simulink model "Lab_5"  (Simulink 9.2)
settings: Solver=VariableStepAuto  StartTime=0.0  StopTime=simulation_time  MaxStep=0.1
values from neighbouring files (symbols this model uses):
  a = (r_a + r_p)/2    (= 7178)    [main.m]
  A_BN_0 = eye(3)    [main.m]
  A_i = [A_i_1, A_i_2, A_i_3]    [main.m]
  alpha_m = deg2rad(11)    [main.m]
  C_d = 2.2    [main.m]
  dim = [w, l, h]    [main.m]
  epsilon = deg2rad(23.439)    [main.m]
  i = 40    [main.m]
  I = [I_1,   0,  0 ... (first row only)    [main.m]
  I_inv = inv(I)    [main.m]
  k_d = -0.001    [main.m]
  k_p = -0.001    [main.m]
  m_m = (a_m^3*H_0)*(4*pi/mu_0)    [main.m]
  mu = 398600    [main.m]
  n = 2*pi/(60*60*24*365)    (= 1.99238499086e-07)    [main.m]
  nadir_vector = [1; 0; 0]    [main.m]
  OMG = 0    [main.m]
  omg = 0    [main.m]
  phi_0 = 0    [main.m]
  psi_0 = 0    [main.m]
  Q_C = [ q_c(4)  q_c(3)  -q_c(2) -q_c(1) ... (first row only)    [main.m]
  R_e = 6.378e+03    (= 6378)    [main.m]
  rho_d = 0.1    [main.m]
  rho_s = 0.5    [main.m]
  theta = 0    [main.m]
  theta_0 = 0    [main.m]
  w_0 = [w1_0,w2_0,w3_0]    [main.m]
  w_e = [0 0 0.00007291]    [main.m]
undefined symbols (not defined in the file or in its folder): q_0
libraries: sharedtransform x2, vrlib x2, sharedutil x2
settings Model: Creator=fcuzzocrea  LastModifiedBy=fcuzzocrea
settings DataIOCC: LimitDataPoints=off  SaveFormat=Dataset  SignalLoggingSaveFormat=Dataset
settings OptimizationCC: LifeSpan=auto
settings DebuggingCC: UnderspecifiedInitializationDetection=Simplified  MergeDetectMultiDrivingBlocksExec=error  FcnCallInpInsideContextMsg=error  StateNameClashWarn=none  LibraryContextMissingDiagnostic=none  SFUnexpectedBacktrackingDiag=error  SFNoUnconditionalDefaultTransitionDiag=error  SFExecutionAtInitializationDiag=warning
settings HardwareCC: ProdBitPerPointer=64  ProdBitPerSizeT=64  ProdBitPerPtrDiffT=64  ProdLargestAtomicFloat=Float  ProdIntDivRoundTo=Zero  ProdEndianess=LittleEndian  ProdWordSize=64  ProdHWDeviceType=Intel->x86-64 (Windows64)
settings ModelReferenceCC: PropagateSignalLabelsOutOfModel=on
settings CodeAppCC: StateflowObjectComments=off
settings GRTTargetCC: TargetLangStandard=C99 (ISO)  GeneratePreprocessorConditionals=Use local settings  CombineOutputUpdateFcns=on  GRTInterface=off
settings ConfigComp: CovMetricSettings=dwe  CovHtmlReporting=off  CovSaveCumulativeToWorkspaceVar=off  CovSaveSingleToWorkspaceVar=off  CovExternalEMLEnable=on

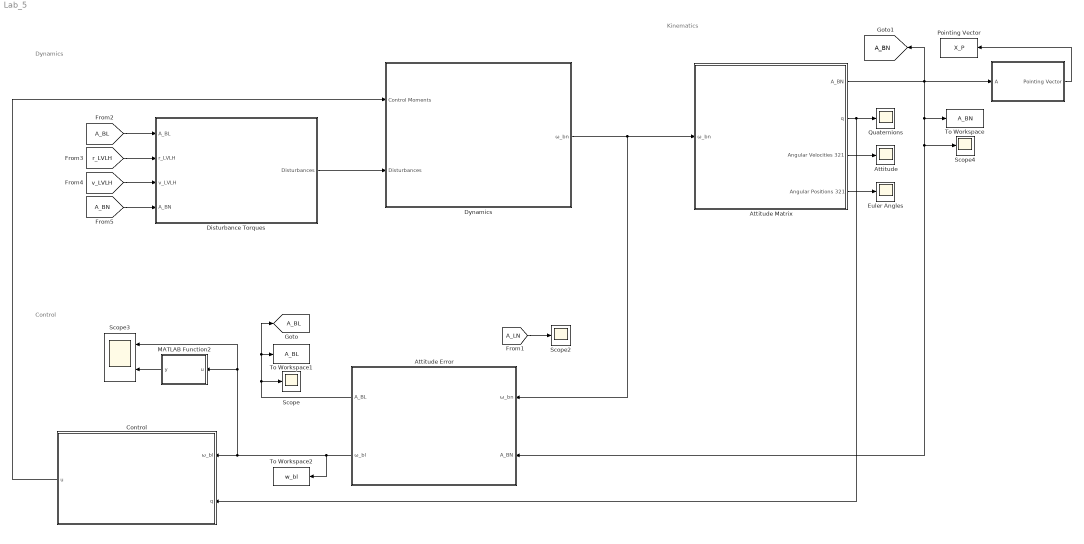
== system Lab_5 ==
  note: Dynamics
  note: Kinematics
  note: Control
  " " : Subsystem
  Attitude : Scope
  Attitude Error : Subsystem
  Attitude Matrix : Subsystem
  Control : Subsystem
  Disturbance Torques : Subsystem
  "Dynamics  " : Subsystem
  Euler Angles : Scope
  MATLAB Function2 : MATLAB Function  TreatAsAtomicUnit=on
  Pointing Vector : ToWorkspace  VariableName=X_P  SampleTime=-1
  Quaternions : Scope
  Scope : Scope
  Scope2 : Scope
  Scope3 : Scope  NumInputPorts=2
  Scope4 : Scope
  To Workspace : ToWorkspace  VariableName=A_BN  SampleTime=-1
  To Workspace1 : ToWorkspace  VariableName=A_BL  SampleTime=-1
  To Workspace2 : ToWorkspace  VariableName=w_bl  SampleTime=-1
  tag scope: A_BL=global, A_BN=global
  wires:
  Disturbance Torques/1(Disturbances) -> "Dynamics  "/2("Disturbances ")
  [r_LVLH] -> Disturbance Torques/2(r_LVLH)
  Attitude Error/1(A_BL) -> [A_BL], To Workspace1/1, Scope/1
  [A_BN] -> Disturbance Torques/4(A_BN)
  Control/1(u) -> "Dynamics  "/1(Control Moments)
  [A_BL] -> Disturbance Torques/1(A_BL)
  " "/1("Pointing Vector ") -> Pointing Vector/1
  Attitude Matrix/3(Angular Velocities 321) -> Attitude/1
  MATLAB Function2/1(y) -> Scope3/2
  [v_LVLH] -> Disturbance Torques/3(v_LVLH)
  Attitude Matrix/2(q) -> Quaternions/1, Control/2(q)
  Attitude Matrix/4(Angular Positions 321) -> Euler Angles/1
  [A_LN] -> Scope2/1
  Attitude Error/2(ω_bl) -> Control/1(ω_bl), Scope3/1, MATLAB Function2/1(u), To Workspace2/1
  Attitude Matrix/1(A_BN) -> Scope4/1, Attitude Error/2(A_BN), To Workspace/1, " "/1(A), [A_BN]
  "Dynamics  "/1(ω_bn) -> Attitude Error/1(ω_bn), Attitude Matrix/1(ω_bn)

== system Lab_5/  ==
  A : Inport
  Constant3 : Constant  Value=[1; 0; 0]  VectorParams1D=off
  Math Function : Math  Operator=transpose  SaturateOnIntegerOverflow=on
  Product1 : Product  Multiplication=Matrix(*)
  "Pointing Vector " : Outport
  wires:
  Constant3/1 -> Product1/2
  Math Function/1 -> Product1/1
  A/1 -> Math Function/1
  Product1/1 -> "Pointing Vector "/1

== system Lab_5/Attitude Error ==
  ω_bn : Inport
  A_BN : Inport  Port=2
  Angular velocity of the  orbital pointing  frame : Subsystem
  Attitude Error : Subsystem
  Body\LVLH Difference : Subsystem
  A_BL : Outport
  ω_bl : Outport  Port=2
  wires:
  ω_bn/1 -> Attitude Error/1(ω_bn)
  A_BN/1 -> Body\LVLH Difference/1("A_BN ")
  Body\LVLH Difference/1("A_BL   ") -> A_BL/1, Attitude Error/2("A_BL ")
  Angular velocity of the  orbital pointing  frame/1(ω_ln) -> Attitude Error/3("ω_ln ")
  Attitude Error/1(ω_bl) -> ω_bl/1

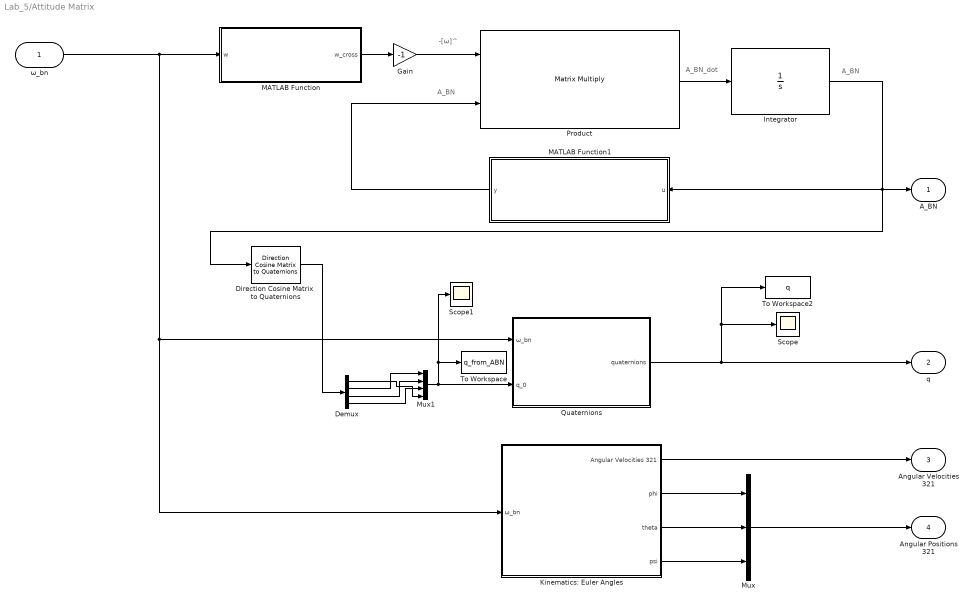
== system Lab_5/Attitude Matrix ==
  note: -[ω]^
  note: A_BN_dot
  note: A_BN
  note: A_BN
  ω_bn : Inport  Unit=rad/s  PortDimensions=3
  Demux : Demux
  Direction Cosine Matrix  to Quaternions : sharedtransform/Direction Cosine Matrix  to Quaternions  aMode=0  action=None  tolerance=eps(2)
      settings: SourceProductName=Aerospace Blockset  SourceProductBaseCode=AE
  Gain : Gain  Gain=-1
  Integrator : Integrator  InitialCondition=A_BN_0
  Kinematics: Euler Angles : Subsystem
  MATLAB Function : MATLAB Function  TreatAsAtomicUnit=on
  MATLAB Function1 : MATLAB Function  TreatAsAtomicUnit=on
  Mux : Mux  Inputs=3
  Mux1 : Mux
  Product : Product  Multiplication=Matrix(*)
  Quaternions : Subsystem
  Scope : Scope
  Scope1 : Scope
  To Workspace : ToWorkspace  VariableName=q_from_ABN  SampleTime=-1
  To Workspace2 : ToWorkspace  VariableName=q  SampleTime=-1
  A_BN : Outport
  q : Outport  Port=2
  Angular Velocities 321 : Outport  Port=3
  Angular Positions 321 : Outport  Port=4
  wires:
  Product/1 -> Integrator/1
  Integrator/1 -> MATLAB Function1/1(u), Direction Cosine Matrix  to Quaternions/1, A_BN/1
  MATLAB Function/1(w_cross) -> Gain/1
  MATLAB Function1/1(y) -> Product/2
  ω_bn/1 -> Quaternions/1(ω_bn), Kinematics: Euler Angles/1(ω_bn), MATLAB Function/1(w)
  Kinematics: Euler Angles/1(Angular Velocities 321) -> Angular Velocities 321/1
  Kinematics: Euler Angles/3(theta) -> Mux/2
  Mux/1 -> Angular Positions 321/1
  Kinematics: Euler Angles/4(psi) -> Mux/3
  Kinematics: Euler Angles/2(phi) -> Mux/1
  Gain/1 -> Product/1
  Mux1/1 -> Quaternions/2("q_0 "), To Workspace/1, Scope1/1
  Quaternions/1(quaternions) -> q/1, Scope/1, To Workspace2/1
  Demux/1 -> Mux1/4
  Demux/2 -> Mux1/1
  Demux/3 -> Mux1/2
  Demux/4 -> Mux1/3
  Direction Cosine Matrix  to Quaternions/1 -> Demux/1

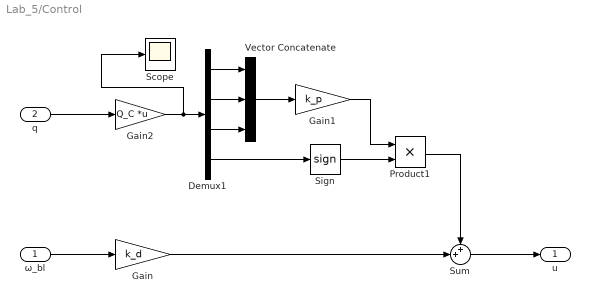
== system Lab_5/Control ==
  ω_bl : Inport
  q : Inport  Port=2
  Demux1 : Demux
  Gain : Gain  Gain=k_d
  Gain1 : Gain  Gain=k_p
  Gain2 : Gain  Gain=Q_C  Multiplication=Matrix(K*u)
  Product1 : Product
  Scope : Scope
  Sign : Signum
  Sum : Sum  Inputs=++|
  Vector Concatenate : Concatenate  NumInputs=3
  u : Outport
  wires:
  ω_bl/1 -> Gain/1
  q/1 -> Gain2/1
  Sum/1 -> u/1
  Demux1/4 -> Sign/1
  Demux1/1 -> Vector Concatenate/1
  Demux1/2 -> Vector Concatenate/2
  Demux1/3 -> Vector Concatenate/3
  Vector Concatenate/1 -> Gain1/1
  Gain1/1 -> Product1/1
  Sign/1 -> Product1/2
  Product1/1 -> Sum/1
  Gain/1 -> Sum/2
  Gain2/1 -> Scope/1, Demux1/1

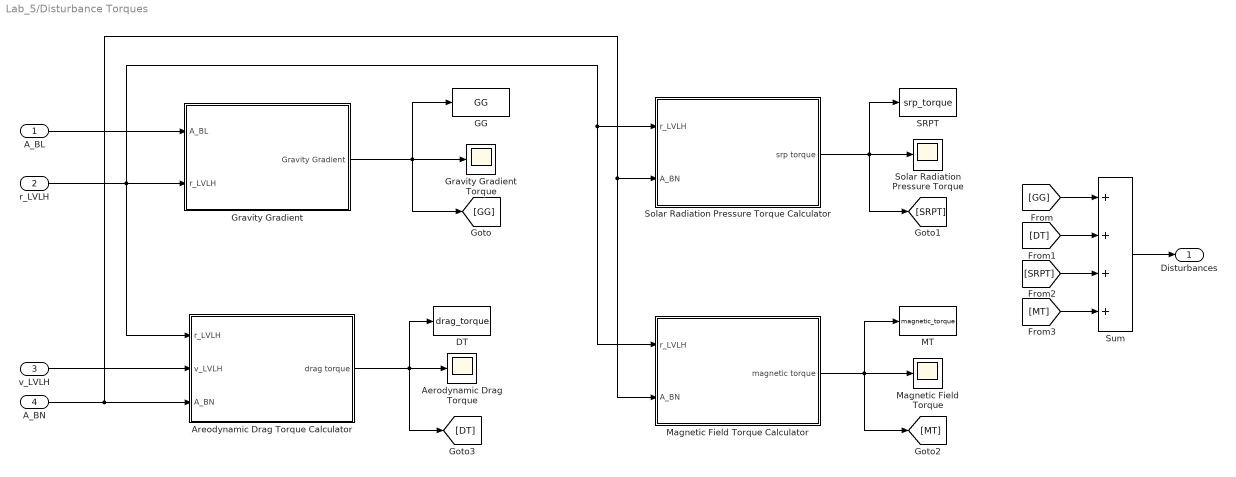
== system Lab_5/Disturbance Torques ==
  A_BL : Inport
  r_LVLH : Inport  Port=2
  v_LVLH : Inport  Port=3
  A_BN : Inport  Port=4
  Aerodynamic Drag Torque : Scope
  "Areodynamic Drag Torque Calculator " : Subsystem
  DT : ToWorkspace  VariableName=drag_torque  SampleTime=-1
  GG : ToWorkspace  VariableName=GG  SampleTime=-1
  Gravity Gradient : Subsystem
  "Gravity Gradient Torque " : Scope
  MT : ToWorkspace  VariableName=magnetic_torque  SampleTime=-1
  Magnetic Field Torque : Scope
  Magnetic Field Torque Calculator : Subsystem
  SRPT : ToWorkspace  VariableName=srp_torque  SampleTime=-1
  Solar Radiation Pressure Torque : Scope
  Solar Radiation Pressure Torque Calculator : Subsystem
  Sum : Sum  Inputs=++++
  Disturbances : Outport
  wires:
  A_BL/1 -> Gravity Gradient/1(A_BL)
  Gravity Gradient/1(Gravity Gradient) -> GG/1, "Gravity Gradient Torque "/1, [GG]
  v_LVLH/1 -> "Areodynamic Drag Torque Calculator "/2(v_LVLH)
  A_BN/1 -> Magnetic Field Torque Calculator/2(A_BN), Solar Radiation Pressure Torque Calculator/2(A_BN), "Areodynamic Drag Torque Calculator "/3(A_BN)
  "Areodynamic Drag Torque Calculator "/1("drag torque ") -> [DT], DT/1, Aerodynamic Drag Torque/1
  Solar Radiation Pressure Torque Calculator/1("srp torque ") -> [SRPT], SRPT/1, Solar Radiation Pressure Torque/1
  Magnetic Field Torque Calculator/1("magnetic torque ") -> [MT], MT/1, Magnetic Field Torque/1
  r_LVLH/1 -> Magnetic Field Torque Calculator/1(r_LVLH), Solar Radiation Pressure Torque Calculator/1(r_LVLH), Gravity Gradient/2(r_LVLH), "Areodynamic Drag Torque Calculator "/1(r_LVLH)
  Sum/1 -> Disturbances/1
  [GG] -> Sum/1
  [DT] -> Sum/2
  [SRPT] -> Sum/3
  [MT] -> Sum/4

== system Lab_5/Dynamics   ==
  Control Moments : Inport
  "Disturbances " : Inport  Port=2
  3x3 Cross Product1 : sharedutil/3x3 Cross Product  aMode=aMode
      settings: SourceProductBaseCode=AE
  Inertia1 : Gain  Gain=I  Multiplication=Matrix(K*u)
  Integrator1 : Integrator  InitialCondition=w_0
  Inverse of inertia tensor1 : Gain  Gain=I_inv  Multiplication=Matrix(K*u)
  Sum : Sum  Inputs=++-
  ω_bn : Outport
  wires:
  Inertia1/1 -> 3x3 Cross Product1/2  "In*ω_b"
  Inverse of inertia tensor1/1 -> Integrator1/1  "ω_b_dot"
  3x3 Cross Product1/1 -> Sum/3  "(In*ω_b)Xω_b"
  Integrator1/1 -> Inertia1/1, 3x3 Cross Product1/1, ω_bn/1  "ω_b"
  Sum/1 -> Inverse of inertia tensor1/1
  Control Moments/1 -> Sum/1
  "Disturbances "/1 -> Sum/2

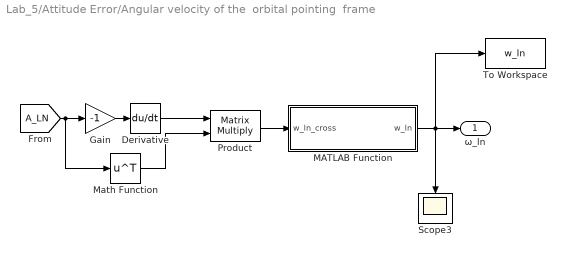
== system Lab_5/Attitude Error/Angular velocity of the  orbital pointing  frame ==
  Derivative : Derivative
  Gain : Gain  Gain=-1
  MATLAB Function : MATLAB Function  TreatAsAtomicUnit=on
  Math Function : Math  Operator=transpose  SaturateOnIntegerOverflow=on
  Product : Product  Multiplication=Matrix(*)
  Scope3 : Scope
  To Workspace : ToWorkspace  VariableName=w_ln  SampleTime=-1
  ω_ln : Outport
  wires:
  Math Function/1 -> Product/2
  Derivative/1 -> Product/1
  Product/1 -> MATLAB Function/1(w_ln_cross)
  MATLAB Function/1(w_ln) -> To Workspace/1, ω_ln/1, Scope3/1
  [A_LN] -> Gain/1, Math Function/1
  Gain/1 -> Derivative/1

== system Lab_5/Attitude Error/Attitude Error ==
  ω_bn : Inport
  "A_BL " : Inport  Port=2
  "ω_ln " : Inport  Port=3
  Product : Product  Multiplication=Matrix(*)
  Subtract : Sum  Inputs=+-
  ω_bl : Outport
  wires:
  Product/1 -> Subtract/2
  Subtract/1 -> ω_bl/1
  ω_bn/1 -> Subtract/1
  "A_BL "/1 -> Product/1
  "ω_ln "/1 -> Product/2

== system Lab_5/Attitude Error/Body\LVLH Difference ==
  "A_BN " : Inport
  LVLH : Subsystem
  Math Function1 : Math  Operator=transpose  SaturateOnIntegerOverflow=on
  Product : Product  Multiplication=Matrix(*)
  "A_BL   " : Outport
  wires:
  "A_BN "/1 -> Product/1
  Product/1 -> "A_BL   "/1
  Math Function1/1 -> Product/2
  LVLH/1("A_LN ") -> Math Function1/1

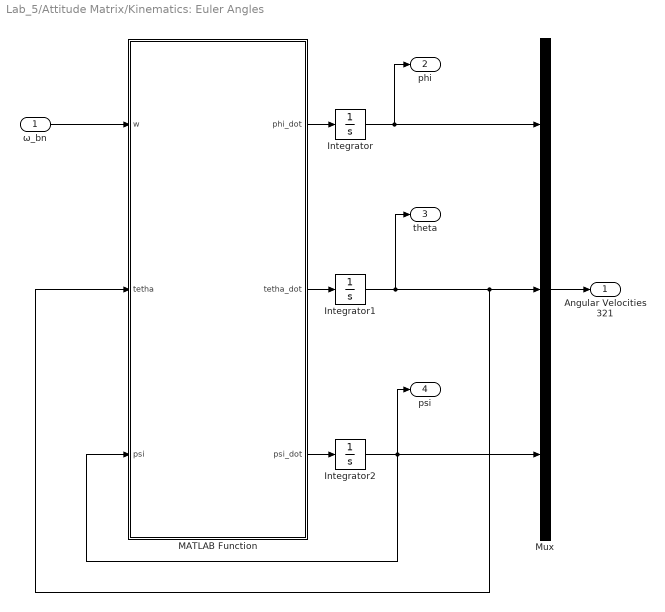
== system Lab_5/Attitude Matrix/Kinematics: Euler Angles ==
  ω_bn : Inport
  Integrator : Integrator  InitialCondition=phi_0
  Integrator1 : Integrator  InitialCondition=theta_0
  Integrator2 : Integrator  InitialCondition=psi_0
  MATLAB Function : MATLAB Function  TreatAsAtomicUnit=on
  Mux : Mux  Inputs=3
  Angular Velocities 321 : Outport
  phi : Outport  Port=2
  theta : Outport  Port=3
  psi : Outport  Port=4
  wires:
  Integrator2/1 -> MATLAB Function/3(psi), Mux/3, psi/1
  Mux/1 -> Angular Velocities 321/1
  Integrator1/1 -> MATLAB Function/2(tetha), Mux/2, theta/1
  Integrator/1 -> Mux/1, phi/1
  MATLAB Function/3(psi_dot) -> Integrator2/1
  MATLAB Function/2(tetha_dot) -> Integrator1/1
  MATLAB Function/1(phi_dot) -> Integrator/1
  ω_bn/1 -> MATLAB Function/1(w)

== system Lab_5/Attitude Matrix/Quaternions ==
  ω_bn : Inport
  "q_0 " : Inport  Port=2
  Integrator2 : Integrator  InitialConditionSource=external  InitialCondition=q_0
  Quaternion Kinematics : MATLAB Function  TreatAsAtomicUnit=on
  quaternions : Outport
  wires:
  Integrator2/1 -> Quaternion Kinematics/1(q), quaternions/1  "q"
  Quaternion Kinematics/1(q_dot) -> Integrator2/1  "dq"
  ω_bn/1 -> Quaternion Kinematics/2(omega)  "ω_b"
  "q_0 "/1 -> Integrator2/2

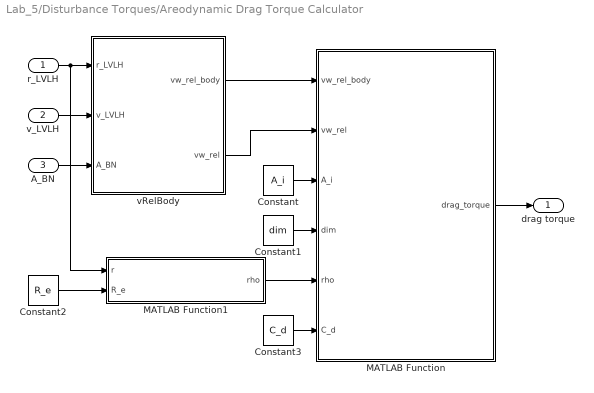
== system Lab_5/Disturbance Torques/Areodynamic Drag Torque Calculator  ==
  r_LVLH : Inport
  v_LVLH : Inport  Port=2
  A_BN : Inport  Port=3
  Constant : Constant  Value=A_i
  Constant1 : Constant  Value=dim
  Constant2 : Constant  Value=R_e
  Constant3 : Constant  Value=C_d
  MATLAB Function : MATLAB Function  TreatAsAtomicUnit=on
  MATLAB Function1 : MATLAB Function  TreatAsAtomicUnit=on
  vRelBody : Subsystem
  "drag torque " : Outport
  wires:
  r_LVLH/1 -> MATLAB Function1/1(r), vRelBody/1(r_LVLH)
  v_LVLH/1 -> vRelBody/2(v_LVLH)
  A_BN/1 -> vRelBody/3(A_BN)
  vRelBody/1(vw_rel_body) -> MATLAB Function/1(vw_rel_body)
  Constant/1 -> MATLAB Function/3(A_i)
  Constant1/1 -> MATLAB Function/4(dim)
  Constant3/1 -> MATLAB Function/6(C_d)
  Constant2/1 -> MATLAB Function1/2(R_e)
  MATLAB Function1/1(rho) -> MATLAB Function/5(rho)
  MATLAB Function/1(drag_torque) -> "drag torque "/1
  vRelBody/2(vw_rel) -> MATLAB Function/2(vw_rel)

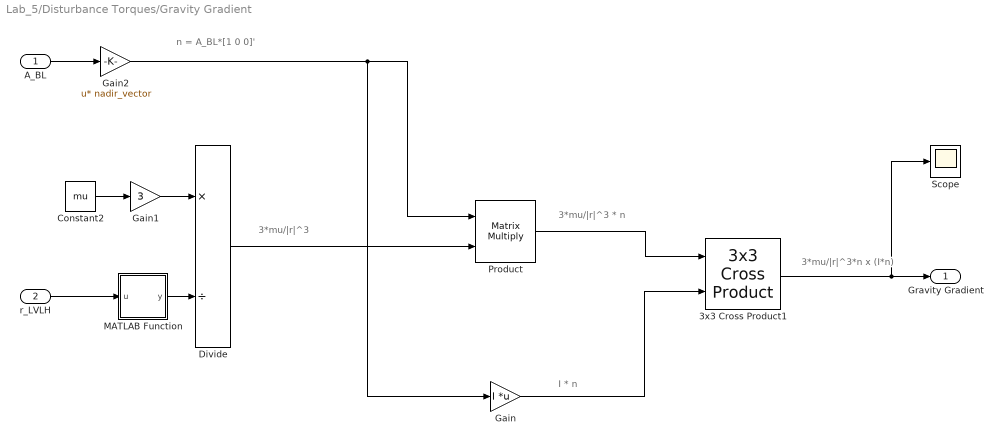
== system Lab_5/Disturbance Torques/Gravity Gradient ==
  note: 3*mu/|r|^3*n x (I*n)
  note: I * n
  note: 3*mu/|r|^3 * n
  note: n = A_BL*[1 0 0]'
  note: 3*mu/|r|^3
  A_BL : Inport
  r_LVLH : Inport  Port=2
  3x3 Cross Product1 : sharedutil/3x3 Cross Product  aMode=aMode
      settings: SourceProductBaseCode=AE
  Constant2 : Constant  Value=mu
  Divide : Product  Inputs=*/
  Gain : Gain  Gain=I  Multiplication=Matrix(K*u)
  Gain1 : Gain  Gain=3
  Gain2 : Gain  Gain=nadir_vector  Multiplication=Matrix(u*K)
  MATLAB Function : MATLAB Function  TreatAsAtomicUnit=on
  Product : Product  Multiplication=Matrix(*)
  Scope : Scope
  Gravity Gradient : Outport
  wires:
  A_BL/1 -> Gain2/1
  r_LVLH/1 -> MATLAB Function/1(u)
  Constant2/1 -> Gain1/1
  Divide/1 -> Product/2
  Product/1 -> 3x3 Cross Product1/1
  Gain/1 -> 3x3 Cross Product1/2
  Gain2/1 -> Gain/1, Product/1
  3x3 Cross Product1/1 -> Gravity Gradient/1, Scope/1
  Gain1/1 -> Divide/1
  MATLAB Function/1(y) -> Divide/2

== system Lab_5/Disturbance Torques/Magnetic Field Torque Calculator ==
  r_LVLH : Inport
  A_BN : Inport  Port=2
  Cross Product : vrlib/Utilities/Cross Product
      settings: SourceProductBaseCode=VR
  Dipole Orientation : Subsystem
  Magnetic Field : Subsystem
  Product : Product  Multiplication=Matrix(*)
  Scope4 : Scope
  "magnetic torque " : Outport
  wires:
  r_LVLH/1 -> Magnetic Field/1(r)
  A_BN/1 -> Product/1
  Product/1 -> Cross Product/1
  Cross Product/1 -> "magnetic torque "/1
  Magnetic Field/1("B ") -> Scope4/1, Product/2
  Dipole Orientation/1(m) -> Cross Product/2, Magnetic Field/2(m)

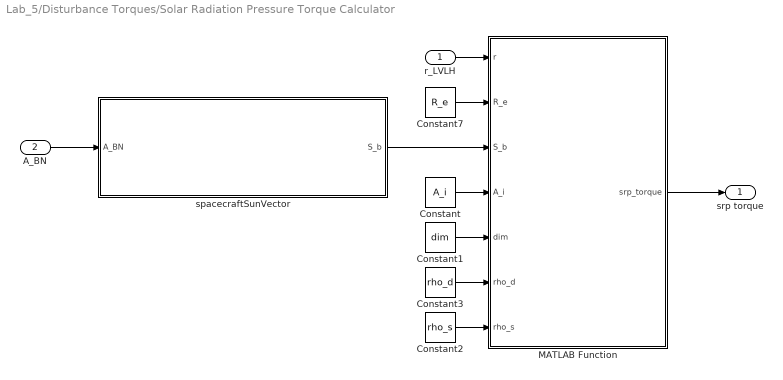
== system Lab_5/Disturbance Torques/Solar Radiation Pressure Torque Calculator ==
  r_LVLH : Inport
  A_BN : Inport  Port=2
  Constant : Constant  Value=A_i
  Constant1 : Constant  Value=dim
  Constant2 : Constant  Value=rho_s
  Constant3 : Constant  Value=rho_d
  Constant7 : Constant  Value=R_e
  MATLAB Function : MATLAB Function  TreatAsAtomicUnit=on
  spacecraftSunVector : Subsystem
  "srp torque " : Outport
  wires:
  A_BN/1 -> spacecraftSunVector/1(A_BN)
  spacecraftSunVector/1("S_b ") -> MATLAB Function/3(S_b)
  Constant/1 -> MATLAB Function/4(A_i)
  Constant1/1 -> MATLAB Function/5(dim)
  Constant3/1 -> MATLAB Function/6(rho_d)
  Constant2/1 -> MATLAB Function/7(rho_s)
  r_LVLH/1 -> MATLAB Function/1(r)
  Constant7/1 -> MATLAB Function/2(R_e)
  MATLAB Function/1(srp_torque) -> "srp torque "/1

== system Lab_5/Attitude Error/Body\LVLH Difference/LVLH ==
  Demux : Demux
  Direction Cosine Matrix  to Quaternions : sharedtransform/Direction Cosine Matrix  to Quaternions  aMode=0  action=None  tolerance=eps(2)
      settings: SourceProductName=Aerospace Blockset  SourceProductBaseCode=AE
  Full Orbital Dynamics : Subsystem
  Initial Conditions (KEP) : Constant  Value=[a, e, i, OMG, omg, theta]
  Mux1 : Mux
  Planetary Constant : Constant  Value=mu
  To Workspace3 : ToWorkspace  VariableName=q_ALN  SampleTime=-1
  "A_LN " : Outport
  tag scope: A_LN=global
  wires:
  Planetary Constant/1 -> Full Orbital Dynamics/1(mu)
  Initial Conditions (KEP)/1 -> Full Orbital Dynamics/2(Initial Condition (kep))
  Full Orbital Dynamics/1(A_LN) -> Direction Cosine Matrix  to Quaternions/1, [A_LN], "A_LN "/1
  Mux1/1 -> To Workspace3/1
  Demux/3 -> Mux1/2
  Demux/4 -> Mux1/3
  Demux/1 -> Mux1/4
  Demux/2 -> Mux1/1
  Direction Cosine Matrix  to Quaternions/1 -> Demux/1

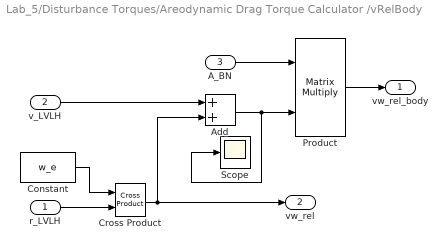
== system Lab_5/Disturbance Torques/Areodynamic Drag Torque Calculator /vRelBody ==
  r_LVLH : Inport
  v_LVLH : Inport  Port=2
  A_BN : Inport  Port=3
  Add : Sum
  Constant : Constant  Value=w_e
  Cross Product : vrlib/Utilities/Cross Product
      settings: SourceProductBaseCode=VR
  Product : Product  Multiplication=Matrix(*)
  Scope : Scope
  vw_rel_body : Outport
  vw_rel : Outport  Port=2
  wires:
  Add/1 -> Scope/1, Product/2
  Constant/1 -> Cross Product/1
  r_LVLH/1 -> Cross Product/2
  Product/1 -> vw_rel_body/1
  v_LVLH/1 -> Add/1
  A_BN/1 -> Product/1
  Cross Product/1 -> vw_rel/1, Add/2

== system Lab_5/Disturbance Torques/Magnetic Field Torque Calculator/Dipole Orientation ==
  Constant : Constant  Value=sin(alpha_m)
  Constant1 : Constant  Value=cos(alpha_m)
  Cosine Wave : Sin  Frequency=w_e(3)  Phase=pi/2  SampleTime=0
  Product : Product
  Product1 : Product
  Sine Wave : Sin  Frequency=w_e(3)  SampleTime=0
  Vector Concatenate : Concatenate  NumInputs=3
  m : Outport
  wires:
  Product/1 -> Vector Concatenate/2
  Vector Concatenate/1 -> m/1
  Cosine Wave/1 -> Product1/2
  Sine Wave/1 -> Product/2
  Constant1/1 -> Vector Concatenate/3
  Product1/1 -> Vector Concatenate/1
  Constant/1 -> Product/1, Product1/1

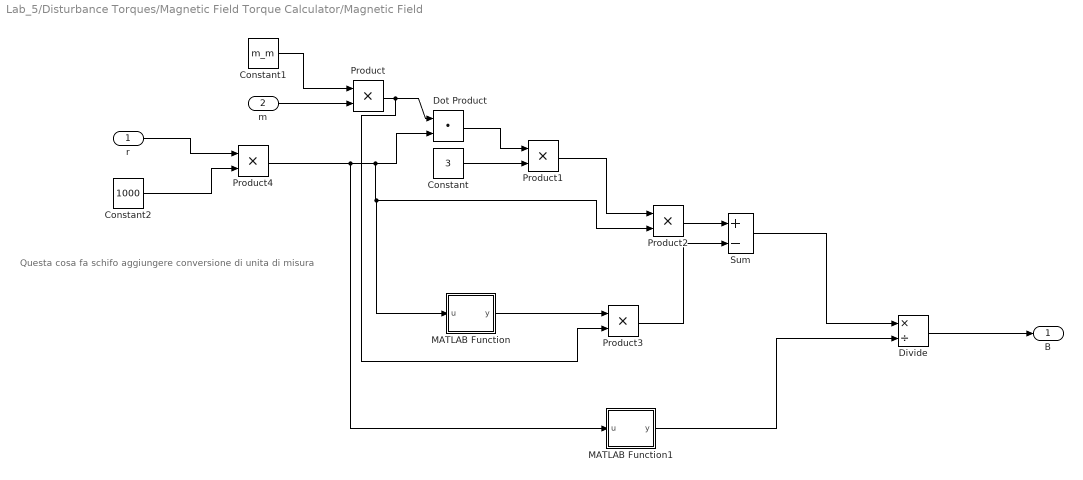
== system Lab_5/Disturbance Torques/Magnetic Field Torque Calculator/Magnetic Field ==
  note: Questa cosa fa schifo aggiungere conversione di unita di misura
  r : Inport  Unit=km
  m : Inport  Port=2
  Constant : Constant  Value=3
  Constant1 : Constant  Value=m_m
  Constant2 : Constant  Value=1000
  Divide : Product  Inputs=*/
  Dot Product : DotProduct  InputSameDT=on  OutDataTypeStr=Inherit: Inherit via internal rule
  MATLAB Function : MATLAB Function  TreatAsAtomicUnit=on
  MATLAB Function1 : MATLAB Function  TreatAsAtomicUnit=on
  Product{,1..4} (5 alike) : Product
  Sum : Sum  Inputs=+-
  "B " : Outport
  wires:
  MATLAB Function1/1(y) -> Divide/2
  Sum/1 -> Divide/1
  Product3/1 -> Sum/2
  MATLAB Function/1(y) -> Product3/1
  Product2/1 -> Sum/1
  Product1/1 -> Product2/1
  Constant/1 -> Product1/2
  Dot Product/1 -> Product1/1
  Product4/1 -> Dot Product/2, Product2/2, MATLAB Function/1(u), MATLAB Function1/1(u)
  Product/1 -> Dot Product/1, Product3/2
  Divide/1 -> "B "/1
  m/1 -> Product/2
  Constant1/1 -> Product/1
  r/1 -> Product4/1
  Constant2/1 -> Product4/2

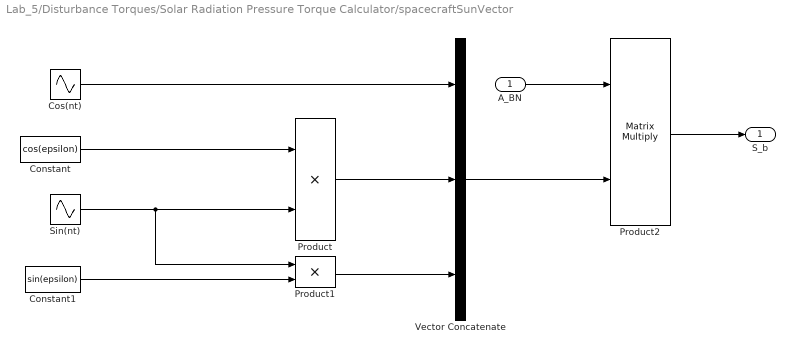
== system Lab_5/Disturbance Torques/Solar Radiation Pressure Torque Calculator/spacecraftSunVector ==
  A_BN : Inport
  Constant : Constant  Value=cos(epsilon)
  Constant1 : Constant  Value=sin(epsilon)
  Cos(nt) : Sin  Frequency=n  Phase=pi/2  SampleTime=0
  Product : Product
  Product1 : Product
  Product2 : Product  Multiplication=Matrix(*)
  Sin(nt) : Sin  Frequency=n  SampleTime=0
  Vector Concatenate : Concatenate  NumInputs=3
  "S_b " : Outport
  wires:
  Product2/1 -> "S_b "/1
  Constant/1 -> Product/1
  Constant1/1 -> Product1/2
  Sin(nt)/1 -> Product1/1, Product/2
  Product1/1 -> Vector Concatenate/3
  Vector Concatenate/1 -> Product2/2
  A_BN/1 -> Product2/1
  Product/1 -> Vector Concatenate/2
  Cos(nt)/1 -> Vector Concatenate/1

== system Lab_5/Attitude Error/Body\LVLH Difference/LVLH/Full Orbital Dynamics ==
  mu : Inport
  Initial Condition (kep) : Inport  Port=2
  "  " : ToWorkspace  VariableName=r_LVLH  SampleTime=-1
  Compute R and V of reference orbit : Subsystem
  MATLAB Function : MATLAB Function  TreatAsAtomicUnit=on
  To Workspace : ToWorkspace  VariableName=A_LN  SampleTime=-1
  A_LN : Outport
  tag scope: r_LVLH=global, v_LVLH=global
  wires:
  mu/1 -> Compute R and V of reference orbit/1(mu)
  Initial Condition (kep)/1 -> Compute R and V of reference orbit/2(Initial Conditions)
  Compute R and V of reference orbit/1(r) -> [r_LVLH], "  "/1, MATLAB Function/1(r)
  MATLAB Function/1(A_LN) -> A_LN/1, To Workspace/1
  Compute R and V of reference orbit/2(r_dot) -> [v_LVLH], MATLAB Function/2(r_dot)

== system Lab_5/Attitude Error/Body\LVLH Difference/LVLH/Full Orbital Dynamics/Compute R and V of reference orbit ==
  mu : Inport
  Initial Conditions : Inport  Port=2
  Initial Position : Subsystem
  Initial Velocity : Subsystem
  Integrator : Integrator  InitialConditionSource=external  InitialCondition=[r,v]=kep2car(kep,mu);  ContinuousStateAttributes='velocity'
  Integrator2 : Integrator  InitialConditionSource=external  InitialCondition=[r,v]=kep2car(kep,mu);  ContinuousStateAttributes='position'
  Orbital Dynamics : MATLAB Function  TreatAsAtomicUnit=on
  r : Outport
  r_dot : Outport  Port=2
  wires:
  Initial Conditions/1 -> Initial Position/2(Initial Conditions), Initial Velocity/2(Initial Conditions)
  Initial Position/1(r_0) -> Integrator2/2
  Initial Velocity/1(r_dot_0) -> Integrator/2
  Orbital Dynamics/1(r_dot_dot) -> Integrator/1
  Integrator/1 -> r_dot/1, Integrator2/1
  mu/1 -> Initial Position/1(mu), Initial Velocity/1(mu), Orbital Dynamics/2(mu)
  Integrator2/1 -> Orbital Dynamics/1(r), r/1

== system Lab_5/Attitude Error/Body\LVLH Difference/LVLH/Full Orbital Dynamics/Compute R and V of reference orbit/Initial Position ==
  mu : Inport
  Initial Conditions : Inport  Port=2
  MATLAB Function2 : MATLAB Function  TreatAsAtomicUnit=on
  r_0 : Outport
  wires:
  MATLAB Function2/1(r_0) -> r_0/1
  mu/1 -> MATLAB Function2/2(mu)
  Initial Conditions/1 -> MATLAB Function2/1(kep)

== system Lab_5/Attitude Error/Body\LVLH Difference/LVLH/Full Orbital Dynamics/Compute R and V of reference orbit/Initial Velocity ==
  mu : Inport
  Initial Conditions : Inport  Port=2
  MATLAB Function1 : MATLAB Function  TreatAsAtomicUnit=on
  r_dot_0 : Outport
  wires:
  MATLAB Function1/1(r_dot_0) -> r_dot_0/1
  mu/1 -> MATLAB Function1/2(mu)
  Initial Conditions/1 -> MATLAB Function1/1(kep)

== matlab function Attitude Matrix/Kinematics: Euler Angles/MATLAB Function ==
  data: phi_dot output double; tetha_dot output double; psi_dot output double; w input double; tetha input double; psi input double
function [phi_dot,tetha_dot, psi_dot] = euler_eqtns(w, tetha, psi)

% Euler rotations (sequence 321)
phi_dot = 1/cos(tetha)*(w(2)*sin(psi) + w(3)*cos(psi));
tetha_dot = (w(2)*cos(psi)-w(3)*sin(psi));
psi_dot = w(1) + 1/cos(tetha)*(w(2)*sin(tetha)*sin(psi) + w(3)*sin(tetha)*cos(psi)); 

end

== matlab function Attitude Matrix/MATLAB Function ==
  data: w input double; w_cross output double
function w_cross  = assembly_w_cross(w)

w_cross = [0, -w(3), w(2);
           w(3), 0, -w(1);
          -w(2), w(1), 0];

== matlab function Attitude Matrix/MATLAB Function1 ==
  data: u input double; y output double
function y = ortonormalize(u)
%#codegen
% Ortonormalize a matrix.
% Reference : Lecture 7, Slide 5 SADC Polimi

y = u.*3/2 - u*u'*(u./2);

y = u;

end

== matlab function Attitude Matrix/Quaternions/Quaternion Kinematics ==
  data: q input double size=4; q_dot output double size=4; omega input double size=3
function q_dot = quat_kin(q, omega)

qnorm = sqrt(q(1)^2 + q(2)^2 + q(3)^2 + q(4)^2);
q = q./qnorm;

W = [ q(4) -q(3)  q(2) ;
      q(3)  q(4) -q(1) ;
     -q(2)  q(1)  q(4) ; 
     -q(1) -q(2) -q(3)];

q_dot = 0.5 * W * omega;

== matlab function Disturbance Torques/Areodynamic Drag Torque Calculator /MATLAB Function ==
  data: vw_rel_body input double; vw_rel input double; drag_torque output double; A_i input double; dim input double; rho input double; C_d input double
function drag_torque   = aerodrag(vw_rel_body,vw_rel,A_i,dim,rho, C_d)

% Velocity is in km/s, we need it in m/s
vw_rel_body = vw_rel_body .* 1e3;

% Define normal vectors
n_1 = [1 0 0];
n_2 = [0 1 0];
n_3 = [0 0 1];
n_4 = [-1 0 0];
n_5 = [0 -1 0];
n_6 = [0 0 -1];

% Dimensions
w = dim(1);
l = dim(2);
h = dim(3);

% Sections
A_i_1 = A_i(1);
A_i_2 = A_i(2);
A_i_3 = A_i(3);
A_i_4 = A_i(1);
A_i_5 = A_i(2);
A_i_6 = A_i(3);

% Distance between the center of pressure and the center of mass 0.1*rcg
r_1 = [h/2 0.1 0.1];
r_2 = [0.2 l/2 0.2];
r_3 = [0.4 0.4 w/2];
r_4 = [-h/2 0.1 0.1];
r_5 = [0.2 -l/2 0.2];
r_6 = [0.4 0.4 -w/2];

% Compute Aerodynamic Torque : reference Fundamentals of Spacecraft
% Dynamics and Control pag. 108
% Compute the dynamic pressure
dynamic_pressure = -0.5*rho*norm(vw_rel)*vw_rel_body;

% Compute torque due to the aerodynamic force only on face wetted by air
% If dot(n_1,vw_rel_body/norm(vw_rel_body)) >=0 then the face is wetted
% othewise no.
if dot(n_1,vw_rel_body/norm(vw_rel)) >= 0
    F_aero_1 = dynamic_pressure * C_d * A_i_1 * dot(n_1,vw_rel_body)/norm(vw_rel);
    T_aero_1 = cross(r_1,F_aero_1);
else
    T_aero_1 = [0 0 0];
end

if dot(n_2,vw_rel_body/norm(vw_rel)) >= 0
    F_aero_2 = dynamic_pressure * C_d * A_i_2 * dot(n_2,vw_rel_body)/norm(vw_rel);
    T_aero_2 = cross(r_2,F_aero_2);
else
    T_aero_2 = [0 0 0];
end

if dot(n_3,vw_rel_body/norm(vw_rel)) >= 0
    F_aero_3 = dynamic_pressure * C_d * A_i_3 * dot(n_3,vw_rel_body)/norm(vw_rel);
    T_aero_3 = cross(r_3,F_aero_3);
else
    T_aero_3 = [0 0 0];
end

if dot(n_4,vw_rel_body/norm(vw_rel)) >= 0
    F_aero_4 = dynamic_pressure * C_d * A_i_4 * dot(n_4,vw_rel_body)/norm(vw_rel);
    T_aero_4 = cross(r_4,F_aero_4);
else
    T_aero_4 = [0 0 0];
end

if dot(n_5,vw_rel_body/norm(vw_rel)) >= 0
    F_aero_5 = dynamic_pressure * C_d * A_i_5 * dot(n_5,vw_rel_body)/norm(vw_rel);
    T_aero_5 = cross(r_5,F_aero_5);
else
    T_aero_5 = [0 0 0];
end

if dot(n_6,vw_rel_body/norm(vw_rel)) >= 0
    F_aero_6 = dynamic_pressure * C_d * A_i_6 * dot(n_6,vw_rel_body)/norm(vw_rel);
    T_aero_6 = cross(r_6,F_aero_6);
else
    T_aero_6 = [0 0 0];
end

% Sum drag on all the surface
drag_torque = [T_aero_1 + T_aero_2 + T_aero_3 + T_aero_4 + T_aero_5 + T_aero_5 + T_aero_6]';

end

== matlab function MATLAB Function2 ==
  data: u input double; y output double
function y = fcn(u)

y = norm(u);

== matlab function Disturbance Torques/Areodynamic Drag Torque Calculator /MATLAB Function1 ==
  data: r input double; rho output double; R_e input double
function rho = density_calculator(r,R_e)
%#codegen
% Exponential model for computing density

h = norm(r') - R_e;


H = 0;
h0 = 0;
rho_0 = 0; 
rho = 0;

if h > 200 && h <= 250
    H = 38.5;
    h0 = 200;
    rho_0 = 2.780e-10;
elseif h > 250 && h <= 300
    H = 46.9;
    h0 = 250;
    rho_0 = 7.248e-11;
elseif h > 300 && h <= 350
    H = 52.5;
    h0 = 300;
    rho_0 = 2.418e-11;
elseif h > 350 && h <= 400
    H = 56.4;
    h0 = 350;
    rho_0 = 9.158e-12;
elseif h > 400 && h <= 450
    H = 59.4;
    h0 = 400;
    rho_0 = 3.725e-12;
elseif h > 450 && h <= 500
    H = 62.2;
    h0 = 450;
    rho_0 = 1.585e-12;
elseif h > 500 && h <= 600
    H = 65.8;
    h0 = 500;
    rho_0 = 6.967e-13;
elseif h > 600 && h <= 700
    H = 79.0;
    h0 = 600;
    rho_0 = 1.454e-13;
elseif h > 700 && h <= 800
    H = 109.0;
    h0 = 700;
    rho_0 = 3.614e-14;
elseif h > 800 && h <= 900
    H = 164.0;
    h0 = 800;
    rho_0 = 1.170e-14;
elseif h >= 900 && h < 1000
    H = 225.0;
    h0 = 900;
    rho_0 = 5.245e-15;
elseif h >= 1000 
    H = 260.0;
    h0 = 1000;
    rho_0 = 3.019e-15;
end

rho = rho_0*exp(-(h-h0)/H);

== matlab function Attitude Error/Angular velocity of the orbital pointing frame/MATLAB Function ==
  data: w_ln_cross input double; w_ln output double
function w_ln = w_component_extractor(w_ln_cross)

w_1 = w_ln_cross(3,2);
w_2 = w_ln_cross(1,3);
w_3 = w_ln_cross(2,1);

w_ln = [w_1, w_2, w_3]';
end

== matlab function Attitude Error/Body\LVLH Difference/LVLH/Full Orbital Dynamics/Compute R and V of reference orbit/Initial Position/MATLAB Function2 ==
  data: r_0 output double; kep input double; mu input double
function r_0  = kep2car(kep,mu)

% Using kep2car function to find position and velocity at initial condition
[r_0,~]=kep2car(kep,mu);

end

== matlab function Attitude Error/Body\LVLH Difference/LVLH/Full Orbital Dynamics/Compute R and V of reference orbit/Initial Velocity/MATLAB Function1 ==
  data: r_dot_0 output double; kep input double; mu input double
function r_dot_0  = kep2car(kep,mu)

% Using kep2car function to find velocity at initial condition
[~,r_dot_0]=kep2car(kep,mu);

end

== matlab function Attitude Error/Body\LVLH Difference/LVLH/Full Orbital Dynamics/Compute R and V of reference orbit/Orbital Dynamics ==
  data: r input double; r_dot_dot output double; mu input double
function r_dot_dot  = orbit_equation(r,mu)

r_dot_dot = -(mu/norm(r)^3)*r;

end

== matlab function Attitude Error/Body\LVLH Difference/LVLH/Full Orbital Dynamics/MATLAB Function ==
  data: r input double; A_LN output double; r_dot input double
function A_LN = assembly_A_LN(r,r_dot)
% This M-Function builds an LVLH frame from a position vector and a 
% velocity vector

r = r';
r_dot = r_dot';

o_1 = - r/norm(r);                                      % Points toward the Earth, aligned with S/C - Earth direction (x)
o_3 = - (cross(r,r_dot))/(norm(cross(r,r_dot)));         % Points in the direction of angular momentum vector (z)
o_2 = cross(o_3,o_1);                                   % Points into the direction of the motion (y)

A_LN = [o_1; o_2; o_3];

end

== matlab function Disturbance Torques/Magnetic Field Torque Calculator/Magnetic Field/MATLAB Function ==
  data: u input double; y output double
function y = norm2(u)

y = (norm(u))^2;

end

== matlab function Disturbance Torques/Magnetic Field Torque Calculator/Magnetic Field/MATLAB Function1 ==
  data: u input double; y output double
function y = norm5(u)

y = (norm(u))^5;

end

== matlab function Disturbance Torques/Solar Radiation Pressure Torque Calculator/MATLAB Function ==
  data: r input double; R_e input double; S_b input double; srp_torque output double; A_i input double; dim input double; rho_d input double; rho_s input double
function srp_torque  = srp(r, R_e, S_b, A_i, dim, rho_d, rho_s)

% Define normal vectors
n_1 = [1 0 0];
n_2 = [0 1 0];
n_3 = [0 0 1];
n_4 = [-1 0 0];
n_5 = [0 -1 0];
n_6 = [0 0 -1];

% Dimensions 
w = dim(1);
l = dim(2);
h = dim(3);

% Sections 
A_i_1 = A_i(1);
A_i_2 = A_i(2);
A_i_3 = A_i(3);
A_i_4 = A_i(1);
A_i_5 = A_i(2);
A_i_6 = A_i(3);

% Distance between the center of pressure and the center of mass
% +0.1*rcg(da aggiungere)
r_1 = [h/2 0.1 0.1];
r_2 = [0.2 l/2 0.2];
r_3 = [0.4 0.4 w/2];
r_4 = [-h/2 0.1 0.1];
r_5 = [0.2 -l/2 0.2];
r_6 = [0.4 0.4 -w/2];

% Compute Solar Radiation Pressure
% Values taken from  Fundamentals of Spacecraft
% Attitude Determination and Control pag. 421
solar_flux = 1362;        % W/m^2
c = 299792458;            % m/s
P = solar_flux/c;         % Pa

S_b = S_b';

% Compute SRP on all the surface only if we are not shadowed by the Earth
if dot(r,S_b) < -sqrt((norm(r))^2 - R_e^2)
    srp_torque = [0 0 0]';
else    
    % Compute torque due to the solar radiation pressure only exposed faces.
    % If dot(S_b,n_i)) => 1 then the face is exposed othewise no.
    if dot(S_b,n_1) >= 0
        F_srp_1 = P*A_i_1*dot(S_b,n_1) * ((1-rho_s)*S_b + (2*rho_s*dot(S_b,n_1)+2/3*rho_d)*n_1);
        T_srp_1 = cross(r_1,F_srp_1);
    else
        T_srp_1 = [0 0 0];
    end
    
    if dot(S_b,n_2) >= 0
        F_srp_2 = P*A_i_2*dot(S_b,n_2) * ((1-rho_s)*S_b + (2*rho_s*dot(S_b,n_2)+2/3*rho_d)*n_2);
        T_srp_2 = cross(r_2,F_srp_2);
    else
        T_srp_2 = [0 0 0];
    end
    
    if dot(S_b,n_3) >= 0
        F_srp_3 = P*A_i_3*dot(S_b,n_3) * ((1-rho_s)*S_b + (2*rho_s*dot(S_b,n_3)+2/3*rho_d)*n_3);
        T_srp_3 = cross(r_3,F_srp_3);
    else
        T_srp_3 = [0 0 0];
    end
    
    if dot(S_b,n_4) >= 0
        F_srp_4 = P*A_i_4*dot(S_b,n_4) * ((1-rho_s)*S_b + (2*rho_s*dot(S_b,n_4)+2/3*rho_d)*n_4);
        T_srp_4 = cross(r_4,F_srp_4);
    else
        T_srp_4 = [0 0 0];
    end
    
    if dot(S_b,n_5) >= 0
        F_srp_5 = P*A_i_5*dot(S_b,n_5) * ((1-rho_s)*S_b + (2*rho_s*dot(S_b,n_5)+2/3*rho_d)*n_5);
        T_srp_5 = cross(r_5,F_srp_5);
    else
        T_srp_5 = [0 0 0];
    end
    
    if dot(S_b,n_6) >= 0
        F_srp_6 = P*A_i_6*dot(S_b,n_6) * ((1-rho_s)*S_b + (2*rho_s*dot(S_b,n_6)+2/3*rho_d)*n_6);
        T_srp_6 = cross(r_6,F_srp_6);
    else
        T_srp_6 = [0 0 0];
    end
    % Compute Solar Radiation Pressure on all surfaces
    srp_torque = [T_srp_1 + T_srp_2 + T_srp_3 + T_srp_4 + T_srp_5 + T_srp_5 + T_srp_6]';
end

end

== matlab function Disturbance Torques/Gravity Gradient/MATLAB Function ==
  data: u input double; y output double
function y  = norm3(u)

y = (norm(u))^3;

end
